simulink model "ex1slidingimp"  (R2025b)
settings: Solver=VariableStepAuto  StartTime=0.0  StopTime=250  RelTol=1e-3
values from neighbouring files (symbols this model uses):
  IJ = inv(J)    [ex1slidingmode.m]    (also in ex4pdcon.m)
  J = diag([10400, 8200, 9200])    [ex1slidingmode.m]    (also in ex4pdcon.m = diag([7300, 7000, 3800]))
  q0 = [0.68438 ... (first row only)    [ex1slidingmode.m]    (also in ex4pdcon.m = [1;0;0;0])
  w0 = [0;0;0]    [ex1slidingmode.m]    (also in ex4pdcon.m)
  wr = [1;0;0]    [ex1slidingmode.m]
libraries: vrlib x1
settings Model: Creator=Esteban  LastModifiedBy=Esteban

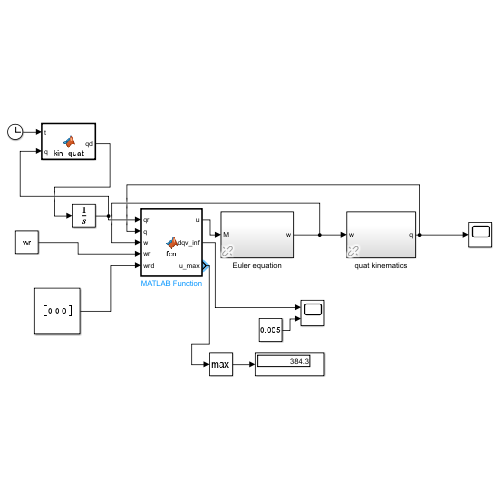
[thumbnail: Simulink's stored preview of the top-level diagram]
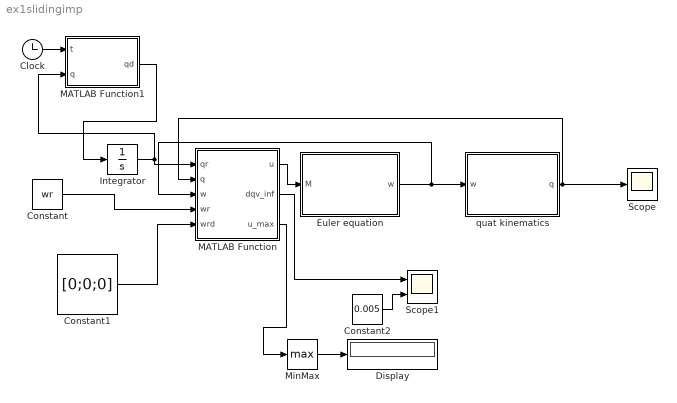
== system ex1slidingimp ==
  Clock : Clock
  Constant : Constant  Value=wr
  Constant1 : Constant  Value=[0;0;0]
  Constant2 : Constant  Value=0.005
  Display : Display
  Euler equation : Subsystem  AncestorBlock=lib_rotations_2014/Euler equation
  Integrator : Integrator  InitialCondition=[1;0;0;0]
  MATLAB Function : MATLAB Function  TreatAsAtomicUnit=on
  MATLAB Function1 : MATLAB Function  TreatAsAtomicUnit=on
  MinMax : MinMax  Function=max
  Scope : Scope
      settings: ActiveDisplayYMinimum=-1  ActiveDisplayYMaximum=1
  Scope1 : Scope  NumInputPorts=2
      settings: ActiveDisplayYMinimum=-1  ActiveDisplayYMaximum=1
  quat kinematics : Subsystem  AncestorBlock=lib_rotations_2014/quat kinematics
  wires:
  Euler equation/1(w) -> MATLAB Function/3(w), quat kinematics/1(w)
  MATLAB Function/1(u) -> Euler equation/1(M)
  quat kinematics/1(q) -> MATLAB Function/2(q), Scope/1
  Clock/1 -> MATLAB Function1/1(t)
  MATLAB Function1/1(qd) -> Integrator/1
  Integrator/1 -> MATLAB Function1/2(q), MATLAB Function/1(qr)
  Constant/1 -> MATLAB Function/4(wr)
  MATLAB Function/2(dqv_inf) -> Scope1/1
  MATLAB Function/3(u_max) -> MinMax/1
  Constant1/1 -> MATLAB Function/5(wrd)
  MinMax/1 -> Display/1
  Constant2/1 -> Scope1/2

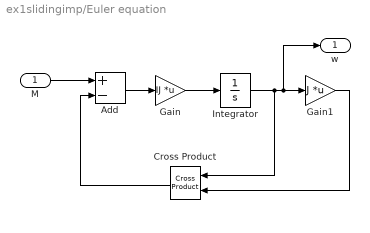
== system ex1slidingimp/Euler equation ==
  M : Inport
  Add : Sum  Inputs=+-
  Cross Product : vrlib/Utilities/Cross Product
  Gain : Gain  Gain=IJ  Multiplication=Matrix(K*u)
  Gain1 : Gain  Gain=J  Multiplication=Matrix(K*u)
  Integrator : Integrator  InitialCondition=w0
  w : Outport  VectorParamsAs1DForOutWhenUnconnected=off
  wires:
  Cross Product/1 -> Add/2
  Add/1 -> Gain/1
  Gain1/1 -> Cross Product/2
  Gain/1 -> Integrator/1
  Integrator/1 -> Gain1/1, w/1, Cross Product/1
  M/1 -> Add/1

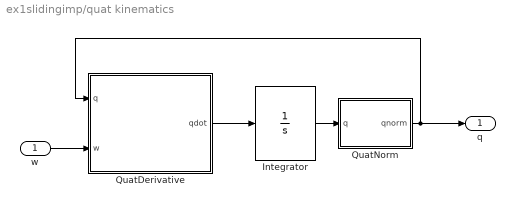
== system ex1slidingimp/quat kinematics ==
  w : Inport  PortDimensions=3
  Integrator : Integrator  InitialCondition=q0
  QuatDerivative : MATLAB Function  TreatAsAtomicUnit=on
  QuatNorm : MATLAB Function  TreatAsAtomicUnit=on
  q : Outport  PortDimensions=4  VectorParamsAs1DForOutWhenUnconnected=off
  wires:
  w/1 -> QuatDerivative/2(w)
  QuatDerivative/1(qdot) -> Integrator/1
  QuatNorm/1(qnorm) -> QuatDerivative/1(q), q/1
  Integrator/1 -> QuatNorm/1(q)

== matlab function ex1slidingimp/quat kinematics/QuatDerivative ==
  data: q input; qdot output; w input
function qdot= QuatDerivative(q,w)
%#codegen
omegaq=[0; w];
Q=[q(1) -q(2) -q(3) -q(4);
    q(2) q(1) -q(4) q(3);
    q(3) q(4) q(1) -q(2);
    q(4) -q(3) q(2) q(1)];
qdot=Q*omegaq/2;

== matlab function ex1slidingimp/quat kinematics/QuatNorm ==
  data: q input; qnorm output
function qnorm = QuatNorm(q)
%#codegen
qnorm=zeros(4,1);
q2=sqrt(q'*q);
qnorm=q/q2;

== matlab function ex1slidingimp/MATLAB Function ==
  data: qr input; q input; w input; u output; wr input; wrd input; dqv_inf output; u_max output
function [u,dqv_inf,u_max] = fcn(qr, q, w, wr, wrd)

J = diag([10400, 8200, 9200]);

k1=89.4337;
k2=0.089474;     
n=178.9474;

dw = wr - w;

qs = [q(1);-q(2:4)];

dq = quatprod(qs,qr);

us = J * (wrd + k2/2 * (dq(1)*dw + cross(dq(2:4),(wr + w)))) + cross(w,J*w);

s = dw + k2*sign(dq(1))*dq(2:4);

u = us + k1*J*tanh(n*s);

dqv_inf = norm(dq(2:4), inf); % Tracks the ||q_tilde||_inf requirement
u_max = norm(u, inf);     % Tracks the max ||u(t)||_inf command effort

== matlab function ex1slidingimp/MATLAB Function1 ==
  data: t input; qd output; q input
function qd=kin_quat(t,q)

w = [1;0;0];

q=q/norm(q);

Q=[-q(2) -q(3) -q(4)
    q(1) -q(4) q(3)
    q(4) q(1)  -q(2)
    -q(3) q(2) q(1)];

qd=1/2*Q*w;
